simulink model "CCToACCFinal1"  (R2025b)
settings: Solver=VariableStepAuto  StartTime=0.0  StopTime=40  RelTol=1e-3
undefined symbols (not defined in the file or in its folder): Cd_air, Cr, default_spacing, m, Sim3dSensor, theta, time_gap, v_set
libraries: drivingscenarioandsensors x5, sim3dautolib x2, sim3dcameralib x1, sim3dlib x1, simulink x1
(part 4 of 4)

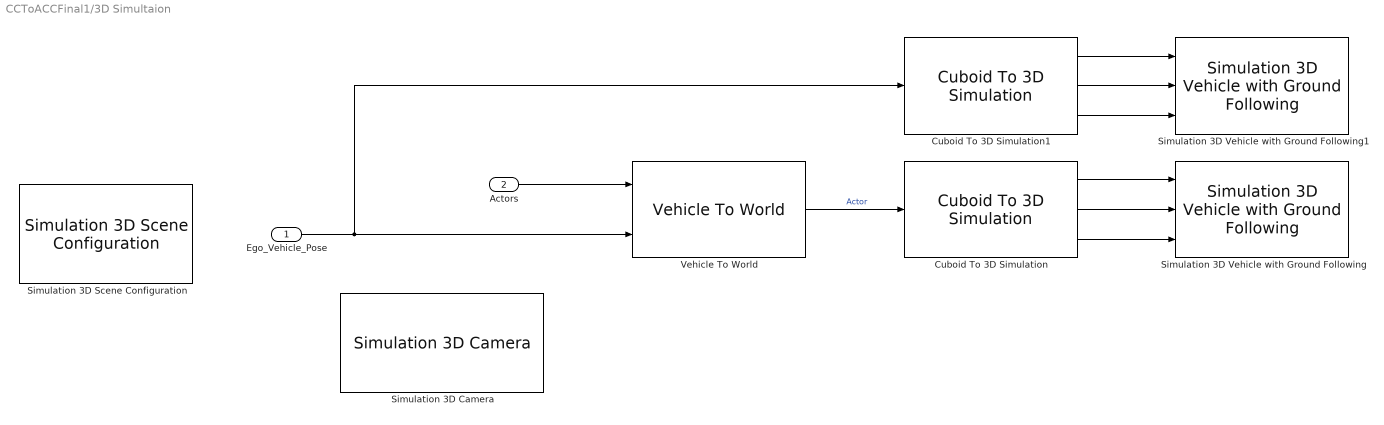
== system CCToACCFinal1/3D Simultaion ==
  Ego_Vehicle_Pose : Inport
  Actors : Inport  Port=2
  Cuboid To 3D Simulation : drivingscenarioandsensors/Cuboid To 3D Simulation  SpecifyActorID=off  ActorIDToConvert=1  SimulateUsing=Interpreted execution
  Cuboid To 3D Simulation1 : drivingscenarioandsensors/Cuboid To 3D Simulation  SpecifyActorID=off  ActorIDToConvert=1  SimulateUsing=Interpreted execution
  Simulation 3D Camera : sim3dcameralib/Simulation 3D Camera  Priority=1  sensorTag=Sim3dSensor�  sensorId=1  sensorName=Sim3dSensor�  vehTagList={'Scene Origin'}  vehTag=Scene Origin  CoordinateSystem=ISO8855  mountLoc=Origin  offsetFlag=off  tmountOffset=[0, 0, 0]  extTmount=off  rmountOffset=[0, 0, 0]  extRmount=off  FocalLength=[1109, 1109]  OpticalCenter=[640, 360]  ImageSize=[720, 1280]  RadialDistortion=[0, 0]  TangentialDistortion=[0, 0]  SensorSkew=0  VisualizeFieldOfView=off  FieldOfViewRange=61  DepthOutportEnabled=off  SemanticOutportEnabled=off  TransformOutportEnabled=off  SampleTime=-1  mountPoint=[0 0 0]  mountOrientation=[0 0 0]  aMode=3  ID=1
      settings: LibrarySourceBlock=drivingsim3d/Simulation 3D Camera
  Simulation 3D Scene Configuration : sim3dlib/Simulation 3D Scene Configuration  Priority=0  ProjectFormat=Default Scenes  SceneDesc=Straight road  ProjectName=C:\Program Files\MATLAB\R2025b\toolbox\shared\sim3d_projects\automotive_project_windows\UE\WindowsNoEditor\VehicleSimulation.exe  ScenePath=/Game/Maps/HwStrght  EnableOpenDRIVE=off  vehTagList={'Custom';'Scene Origin';'SimulinkVehicle1';'SimulinkVehicle2'}  vehTag=SimulinkVehicle2  AttachedCameraRelativeTranslation=[0 0 0]  FreeCameraDefaultInitialTranslation=[-6, 0, 2]  AttachedCameraRelativeRotation=[0 0 0]  FreeCameraDefaultInitialRotation=[0, -15, 0]  ViewpointName=Custom  FreeCameraInitialTranslation=[0, 0, 0]  ViewpointTranslation=[0 0 0]  FreeCameraInitialRotation=[0, 0, 0]  ViewpointRotation=[0 0 0]  OpVisEn=off  Ts=0.1  EnableWindow=on  EnableRemoteAccess=off  EnableWeather=off  SunAzimuth=90  SunAltitude=40.0  EnableGeospatialSun=off  Latitude=0  Longitude=0  Date=2023-01-01  Time=10:30:00  GeoTimeZone=-5.0  SunDaylightSaving=off  wind=1  clouds=10  EnableVolumetricClouds=off  CloudCoverage=0  CloudAltitude=6  fog=0  rain=0  RaindropsEffect=off  SnowDensity=0  EnableGeospatial=off  TilesetSource=Earth terrain  UseTrueOrigin=off  OriginHeight=200  OriginLatitude=40.744652  OriginLongitude=-73.988864  MapStyle=Aerial  AdditionalAssetIDs=[]  UseAdvancedSunSky=off  SolarTime=11  TimeZone=-5  Day=21  Month=9  Year=2022  UseDaylightSavingTime=on  DSTStartDay=10  DSTStartMonth=3  DSTEndDay=3  DSTEndMonth=11  DSTSwitchHour=2  sensorTag=MainCamera1  sensorId=1  sensorName=MainCamera1  mountLoc=Origin  offsetFlag=off  tmountOffset=[0, 0, 0]  rmountOffset=[0, 0, 0]  HorizontalResolution=1280  VerticalResolution=720  HorizontalFOV=60  mountPoint=[0 0 0]  mountOrientation=[0 0 0]  aMode=3  ID=1  GeoTrigger=Inactive  ViewNameList={'Custom'}  ViewTranslationList={'[0 0 0]'}  ViewRotationList={'[0 0 0]'}
      settings: LibrarySourceBlock=drivingsim3d/Simulation 3D Scene Configuration
  Simulation 3D Vehicle with Ground Following : sim3dautolib/Simulation 3D Vehicle with Ground Following  Priority=-1  PassVehMesh=Sport utility vehicle  MeshPath=/MathWorksAutomotiveContent/Vehicles/Muscle/Meshes/SK_MuscleCar.SK_MuscleCar  TrackWidth=1.9  WheelBase=3  WheelRadius=0.35  VehColor=Green  CoordinateSystem=ISO8855  InitialPos=[0, 0, 0]  InitialRot=[0, 0, 0]  ActorName=SimulinkVehicle1  SampleTime=-1  ActorType=SimulinkVehicle  ID=1  aMode=3  ActorTag=SimulinkVehicle1  CoordinateScheme=ISO  VehLightsControl=off  HeadlightColor=[ 1, 1, 1 ]  HighBeamIntensity=100000  LowBeamIntensity=60000  HighBeamConeAngle=70  LowBeamConeAngle=70  LeftHeadlightOrientation=[ 0, 0 ]  RightHeadlightOrientation=[ 0, 0 ]  BrakelightIntensity=500  ReverselightIntensity=500  SignallightIntensity=500  SignallightPeriod=1  SignalPulseWidth=50  TransformOutportEnabled=off
      settings: LibrarySourceBlock=drivingsim3d/Simulation 3D Vehicle with Ground Following
  Simulation 3D Vehicle with Ground Following1 : sim3dautolib/Simulation 3D Vehicle with Ground Following  Priority=-1  PassVehMesh=Muscle car  MeshPath=/MathWorksAutomotiveContent/Vehicles/Muscle/Meshes/SK_MuscleCar.SK_MuscleCar  TrackWidth=1.9  WheelBase=3  WheelRadius=0.35  VehColor=Silver  CoordinateSystem=ISO8855  InitialPos=[0, 0, 0]  InitialRot=[0, 0, 0]  ActorName=SimulinkVehicle2  SampleTime=-1  ActorType=SimulinkVehicle  ID=2  aMode=3  ActorTag=SimulinkVehicle2  CoordinateScheme=ISO  VehLightsControl=off  HeadlightColor=[ 1, 1, 1 ]  HighBeamIntensity=100000  LowBeamIntensity=60000  HighBeamConeAngle=70  LowBeamConeAngle=70  LeftHeadlightOrientation=[ 0, 0 ]  RightHeadlightOrientation=[ 0, 0 ]  BrakelightIntensity=500  ReverselightIntensity=500  SignallightIntensity=500  SignallightPeriod=1  SignalPulseWidth=50  TransformOutportEnabled=off
      settings: LibrarySourceBlock=drivingsim3d/Simulation 3D Vehicle with Ground Following
  Vehicle To World : drivingscenarioandsensors/Vehicle To World  BusNameSource=Auto  BusName=BusVehicleToWorldActors  SimulateUsing=Interpreted execution
  wires:
  Cuboid To 3D Simulation/3 -> Simulation 3D Vehicle with Ground Following/3
  Actors/1 -> Vehicle To World/1
  Cuboid To 3D Simulation/1 -> Simulation 3D Vehicle with Ground Following/1
  Cuboid To 3D Simulation/2 -> Simulation 3D Vehicle with Ground Following/2
  Cuboid To 3D Simulation1/3 -> Simulation 3D Vehicle with Ground Following1/3
  Ego_Vehicle_Pose/1 -> Cuboid To 3D Simulation1/1, Vehicle To World/2
  Vehicle To World/1 -> Cuboid To 3D Simulation/1  "Actor"
  Cuboid To 3D Simulation1/1 -> Simulation 3D Vehicle with Ground Following1/1
  Cuboid To 3D Simulation1/2 -> Simulation 3D Vehicle with Ground Following1/2

== matlab function CCToACCFinal1/MATLAB Function1 ==
  data: v_set input; a_cmd output; default_spacing input; time_gap input; longVelocity input; relDistance input; relVelocity input; v_error output; p_title output; d_safe output
function [a_cmd, v_error, p_title, d_safe] = ACCController( ...
    v_set, default_spacing, time_gap, longVelocity, relDistance, relVelocity)
% ACCController: Adaptive Cruise Control main control law based on the course PDF.
%
%   [a_cmd, v_error, p_title, d_safe] = ACCController( ...
%       v_set, default_spacing, time_gap, longVelocity, relDistance, relVelocity)
%
%   Inputs:
%       v_set           - desired (set) speed of the ego vehicle [m/s]
%       default_spacing - default minimum following distance [m]
%       time_gap        - time gap constant [s]
%       longVelocity    - current longitudinal speed of the ego vehicle [m/s]
%       relDistance     - distance to the lead vehicle [m] (0 means no lead vehicle)
%       relVelocity     - relative speed (ego - lead) [m/s]
%
%   Outputs:
%       a_cmd   - commanded longitudinal acceleration (saturated) [m/s^2]
%       v_error - speed error (v_set - longVelocity) [m/s]
%       p_title - distance error term used inside the controller
%       d_safe  - safe following distance (useful for logging / KPI_block)
%
%   Control law (from PDF):
%       d_safe   = default_spacing + time_gap * longVelocity
%       p_tilde  = d_safe - relDistance
%       u(t)     = k_p * p_tilde + k_v * relVelocity
%
%   Notes:
%       - relVelocity > 0 means the ego vehicle is faster than the lead (closing).
%       - If no lead vehicle is detected (relDistance == 0), the controller uses
%         d_safe as the virtual distance to avoid division by zero or bad behavior.
%       - The final command a_cmd is saturated to physical limits to keep the
%         acceleration within a realistic and comfortable range.

%% --- Controller gains (from PDF, negative due to sign convention) ---
k_p = -0.6;      % distance error gain
k_v = -0.125;    % relative velocity gain

%% --- Speed error (for monitoring only) ---
v_error = v_set - longVelocity;

%% --- Safe following distance ---
% This is the desired distance to the lead vehicle.
d_safe = default_spacing + time_gap * longVelocity;

%% --- Lead vehicle presence ---
% If relDistance is zero, we assume there is no valid lead vehicle.
% In that case, we use d_safe as a virtual distance to avoid distance error jumps.
threshold = 0;  % relDistance == 0 -> no lead
if relDistance > threshold
    distanceUsed = relDistance;
else
    distanceUsed = d_safe;
end

%% --- Distance error term for the controller ---
% p_title (p_tilde) becomes positive if the ego is too close (relDistance < d_safe).
p_title = d_safe - distanceUsed;

%% --- Raw (unsaturated) control law ---
% Combined effect of distance error and relative velocity.
a_cmd_raw = k_p * p_title + k_v * relVelocity;

%% --- Physical saturation of acceleration ---
a_min_phys = -7.5;   % [m/s^2] maximum braking (comfortable/emergency bound)
a_max_phys =  2.0;   % [m/s^2] maximum allowed acceleration

if a_cmd_raw > a_max_phys
    a_cmd = a_max_phys;
elseif a_cmd_raw < a_min_phys
    a_cmd = a_min_phys;
else
    a_cmd = a_cmd_raw;
end

end

== matlab function CCToACCFinal1/MATLAB Function ==
  data: pos input; egoActor output Bus: EgoVehiclePoseBus size=1; vel input; yaw input; yawRate input; egoID input
function egoActor = packEgo(pos,vel,yaw,yawRate,egoID)


egoActor = struct(...
    'ActorID',egoID,...
    'Position', [pos(1) pos(2) 0], ...
    'Velocity', [vel(1) 0 0], ...
    'Roll', 0, ...
    'Pitch', 0, ...
    'Yaw', yaw, ...
    'AngularVelocity', [0 0 yawRate]);

end

== matlab function CCToACCFinal1/MATLAB Function2 ==
  settings: updateMethod=DISCRETE
  data: relDist input; TTC output; relVel input; d_safe input; a input; t input; TTC_min output; viol_rate output; a_max output; a_min output; reset input
function [TTC, TTC_min, viol_rate, a_max, a_min] = ...
    KPI_block(relDist, relVel, d_safe, a, t, reset)
%#codegen

%% --- Persistent variables ---------------------------------------------
persistent TTC_min_p a_max_p a_min_p ...
           follow_time viol_time depth_int ...
           t_prev has_prev

% First call or reset
if isempty(has_prev) || reset > 0
    TTC_min_p   = Inf;
    a_max_p     = -inf;
    a_min_p     =  inf;
    follow_time = 0;
    viol_time   = 0;
    depth_int   = 0;
    t_prev      = t;
    has_prev    = false;
end

% Time step
if ~has_prev
    dt       = 0;
    has_prev = true;
else
    dt = max(t - t_prev, 0);
end
t_prev = t;

%% --- 1) TTC and TTC_min -----------------------------------------------
TTC            = NaN;
TTC_MIN_VALID  = 0.10;
TTC_MAX_VALID  = 20.0;
INTERACTION_K  = 1.5;    % "Critical zone" up to 1.5 times d_safe

if (relDist > 0) && (relVel > 0)
    TTC = relDist / max(relVel, 1e-3);   % Protection against division by zero

    if (TTC > TTC_MIN_VALID) && (TTC < TTC_MAX_VALID) && ...
       (relDist < INTERACTION_K * d_safe)

        if TTC < TTC_min_p
            TTC_min_p = TTC;
        end
    end
end

%% --- 2) FOLLOW time and violation (time + depth) ----------------------
if (relDist > 0) && (dt > 0)
    follow_time = follow_time + dt;

    if relDist < d_safe
        viol_time = viol_time + dt;

        % Normalized depth: 0 .. 1
        depth = (d_safe - relDist) / max(d_safe, 0.1);
        depth = min(max(depth, 0), 1);   % Clamp to [0,1]

        depth_int = depth_int + depth * dt;
    end
end

MIN_FOLLOW_TIME = 1.0;   % [s] if follow time is too short, viol_rate = NaN

if follow_time >= MIN_FOLLOW_TIME
    % If you only want the time ratio:
    % viol_rate = viol_time / follow_time;
    % Full version (time + depth):
    viol_rate = depth_int / follow_time;
else
    viol_rate = NaN;
end

%% --- 3) Acceleration extrema -----------------------------------------
if a > a_max_p
    a_max_p = a;
end
if a < a_min_p
    a_min_p = a;
end
a_max = a_max_p;
a_min = a_min_p;

%% --- 4) TTC_min output ------------------------------------------------
if isinf(TTC_min_p)
    TTC_min = NaN;
else
    TTC_min = TTC_min_p;
end

end

== matlab function CCToACCFinal1/Vehicle Dynamics ==
  data: a_cmd input; a output; v input; m input; Cd_air input; Cr input; theta input
function a = vehicle_dynamics_v2(a_cmd, v, m, Cd_air, Cr, theta)
% VEHICLE_DYNAMICS_V2
% Inputs:
%   a_cmd   : desired longitudinal acceleration from controller [m/s^2]
%   v       : vehicle speed [m/s]
%   m       : mass [kg]
%   Cd_air  : Cd*Af combined coefficient [m^2]
%   Cr      : rolling resistance coefficient [-]
%   theta   : road slope angle [rad] (positive = uphill)
%
% Output:
%   a       : actual longitudinal acceleration [m/s^2]

% --- Constants ---
rho = 1.225;     % air density [kg/m^3]
g   = 9.81;      % gravity [m/s^2]

% --- Physical limits (tune these to your "ego vehicle") ---
P_max        = 80e3;   % max traction power [W]  (e.g., 60kW-120kW typical passenger car)
F_drive_max0 = 4500;   % max drive force cap [N] (torque/traction cap)
F_brake_max0 = 9000;   % max brake force cap [N]
mu           = 0.9;    % tire-road friction (dry asphalt ~0.8-1.0)

% --- Numerical guards ---
m = max(m, 200);          % avoid nonsense masses
v = max(v, 0);            % ACC use-case: forward speed
v_eps = 0.5;              % avoid divide-by-zero in power limit

% --- Resistive forces (oppose motion) ---
% Drag opposes motion ~ v^2
F_drag  = 0.5 * rho * Cd_air * v^2;

% Rolling resistance ~ m*g*Cr (assume forward motion)
F_roll  = m * g * Cr;

% Grade force along road axis ~ m*g*sin(theta)
% theta>0 uphill => positive grade force opposing forward motion
F_grade = m * g * sin(theta);

F_res = F_drag + F_roll + F_grade;

% --- Convert desired acceleration to required traction force ---
% To achieve a_cmd, traction must cover inertia + resistances:
F_req = m * a_cmd + F_res;

% --- Drive/brake limits ---
% Tire friction limit
F_tire_max = mu * m * g;

% Power limit converts to a speed-dependent force limit
F_power_max = P_max / max(v, v_eps);

% Final drive limit
F_drive_max = min([F_drive_max0, F_tire_max, F_power_max]);

% Brake limit (usually friction-limited; keep cap too)
F_brake_max = min(F_brake_max0, F_tire_max);

% Saturate requested force
F_trac = min(max(F_req, -F_brake_max), F_drive_max);

% --- Actual acceleration from net force ---
F_net = F_trac - F_res;
a = F_net / m;

end
